simulink model "b_gaussianNoise"  (R2021a)
settings: Solver=ode1  StartTime=0.0  StopTime=20  FixedStep=integration_step_size  RelTol=1e-3
values from neighbouring files (symbols this model uses):
  Gs = tf(K,[tal 1],'InputDelay',theta)    [list1.m]
libraries: commchan3 x1
settings Model: Creator=Fernando  LastModifiedBy=Fernando

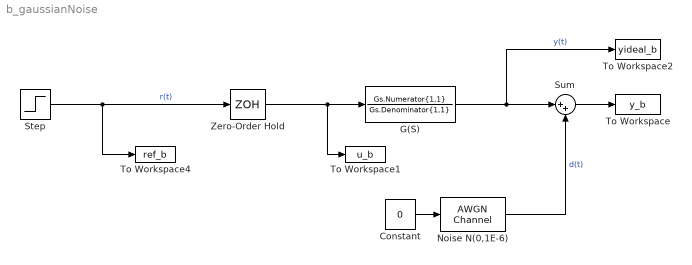
== system b_gaussianNoise ==
  Constant : Constant  Value=0
  G(S) : TransferFcn  Numerator=Gs.Numerator{1,1}  Denominator=Gs.Denominator{1,1}
  Noise N(0,1E-6) : commchan3/AWGN Channel  InputProcessing=Columns as channels (frame based)  seed=67  noiseMode=Variance from mask  EbNodB=10  EsNodB=10  SNRdB=10  bitsPerSym=1  Ps=1  Tsym=1  variance=10^-6
  Step : Step  Time=0  After=0.1  SampleTime=0
  Sum : Sum  Inputs=|++
  To Workspace : ToWorkspace  VariableName=y_b  SaveFormat=Timeseries  SampleTime=-1
      settings: Decimation=100
  To Workspace1 : ToWorkspace  VariableName=u_b  SaveFormat=Timeseries  SampleTime=-1
      settings: Decimation=100
  To Workspace2 : ToWorkspace  VariableName=yideal_b  SaveFormat=Timeseries  SampleTime=-1
      settings: Decimation=100
  To Workspace4 : ToWorkspace  VariableName=ref_b  SaveFormat=Timeseries  SampleTime=-1
      settings: Decimation=100
  Zero-Order Hold : ZeroOrderHold  SampleTime=-1
  wires:
  Zero-Order Hold/1 -> To Workspace1/1, G(S)/1
  Step/1 -> Zero-Order Hold/1, To Workspace4/1  "r(t)"
  G(S)/1 -> To Workspace2/1, Sum/1  "y(t)"
  Sum/1 -> To Workspace/1
  Noise N(0,1E-6)/1 -> Sum/2  "d(t)"
  Constant/1 -> Noise N(0,1E-6)/1
